simulink model "Md62StEnCtrl"  (R2018b)
settings: Solver=FixedStepDiscrete  StartTime=0.0  StopTime=10.0  RelTol=1e-3
undefined symbols (not defined in the file or in its folder): data, KeSMSuFirstRwStBackPosDelta_Val, KeSMSuThrdRwCushFoldPosDelta_Val, KeSMSwAcsMd30PassStFldUpwdDnwdPos1_Val, KeSMSwAcsMd30PassStFrwdBkwdPos1_Val, KeSMSwAcsMd31PassStBkReclnUpwdDnwdPos1_Val, KeSMSwSeatBkLimitPos_Val, KeSMSwSeatBkLimitPosDelt_Val, PassStBkReclnEn_Clear, PassStBkReclnEn_Set, PassStCshnFldEn_Clear, PassStCshnFldEn_Set, PassStFwdBkwdEn_Clear, PassStFwdBkwdEn_Set, SecRwLtStBkReclnEn_Clear, SecRwLtStBkReclnEn_Set, SecRwLtStFwdBkwdEn_Clear, SecRwLtStFwdBkwdEn_Set, SecRwLtStLgrstInwdOtwdEn_Clear, SecRwLtStLgrstInwdOtwdEn_Set, SecRwLtStLgrstUpwdDnwdEn_Clear, SecRwLtStLgrstUpwdDnwdEn_Set, SecRwRtStBkReclnEn_Clear, SecRwRtStBkReclnEn_Set, SecRwRtStFwdBkwdEn_Clear, SecRwRtStFwdBkwdEn_Set, SecRwRtStLgrstInwdOtwdEn_Clear, SecRwRtStLgrstInwdOtwdEn_Set, SecRwRtStLgrstUpwdDnwdEn_Clear, SecRwRtStLgrstUpwdDnwdEn_Set, ThdRwLtStBkReclnEn_Clear, ThdRwLtStBkReclnEn_Set, ThdRwLtStCshnFldEn_Clear, ThdRwLtStCshnFldEn_Set, ThdRwLtStFwdBkwdEn_Clear, ThdRwLtStFwdBkwdEn_Set, ThdRwRtStBkReclnEn_Clear, ThdRwRtStBkReclnEn_Set, ThdRwRtStCshnFldEn_Clear, ThdRwRtStCshnFldEn_Set, ThdRwRtStFwdBkwdEn_Clear, ThdRwRtStFwdBkwdEn_Set, ZeroLEn_Clear, ZeroLEn_Set, ZeroREn_Clear, ZeroREn_Set
libraries: simulink x1
(part 1 of 3)
settings Model: Creator=sn2xws  LastModifiedBy=sn55gm
settings Model: ModifiedHistory=|
  | 25.7.8 V3.13.0 新增Md62
  | 25.7.14 V3.13.1 TrgtPosZone 选择bit位更新
  | 25.7.25 V1.13.3  记忆位置为展开状态，VCU调用mode 61，三排前后电机应和靠背电机一起驱动到目标位置
settings DataIOCC: SaveFormat=StructureWithTime
settings OptimizationCC: DefaultParameterBehavior=Inlined  EnhancedBackFolding=on  PassReuseOutputArgsAs=Individual arguments  ZeroExternalMemoryAtStartup=off  ZeroInternalMemoryAtStartup=off  OptimizeBlockOrder=speed  DifferentSizesBufferReuse=on  OptimizationCustomize=off
settings DebuggingCC: ParameterTunabilityLossMsg=error
settings SFSimCC: MATLABDynamicMemAlloc=off
settings RTWCC: SystemTargetFile=autosar.tlc  GenCodeOnly=on  TemplateMakefile=ert_default_tmf  Description=AUTOSAR  GenerateReport=on  IncludeHyperlinkInReport=on  LaunchReport=on  GenerateTraceInfo=on  GenerateTraceReport=on  GenerateTraceReportSl=on  GenerateTraceReportSf=on  GenerateTraceReportEml=on
settings CodeAppCC: ForceParamTrailComments=on  IgnoreCustomStorageClasses=off  OperatorAnnotations=on  SimulinkDataObjDesc=on  SFDataObjDesc=on  InsertBlockDesc=on
settings STFCustomTargetCC: TargetLangStandard=C99 (ISO)  MultiwordLength=256  ParMdlRefBuildCompliant=on  CompOptLevelCompliant=on  IncludeMdlTerminateFcn=off  CombineOutputUpdateFcns=on  SuppressErrorStatus=on  ERTCustomFileBanners=on  SupportNonFinite=off  SupportComplex=off  SupportContinuousTime=off  SupportNonInlinedSFcns=off  RemoveResetFunc=on  MATLABClassNameForMDSCustomization=Simulink.SoftwareTarget.ERTCustomization  AutosarCompliant=on  UseToolchainInfoCompliant=on  LookupTableObjectStructAxisOrder=2,1,3,4,...  LUTObjectStructOrderEvenSpacing=Size,Table,Breakpoints  SystemTargetFile=autosar.tlc
settings ERTTargetCC: TargetLangStandard=C99 (ISO)  ConcurrentExecutionCompliant=off  IncludeMdlTerminateFcn=off  SuppressErrorStatus=on  SupportNonFinite=off  SupportComplex=off  ModelStepFunctionPrototypeControlCompliant=off  CPPClassGenCompliant=off  AutosarCompliant=on  LookupTableObjectStructAxisOrder=2,1,3,4,...  LUTObjectStructOrderEvenSpacing=Size,Table,Breakpoints  InlinedParameterPlacement=NonHierarchical  ERTCustomFileTemplate=example_file_process.tlc  ERTFilePackagingFormat=Compact

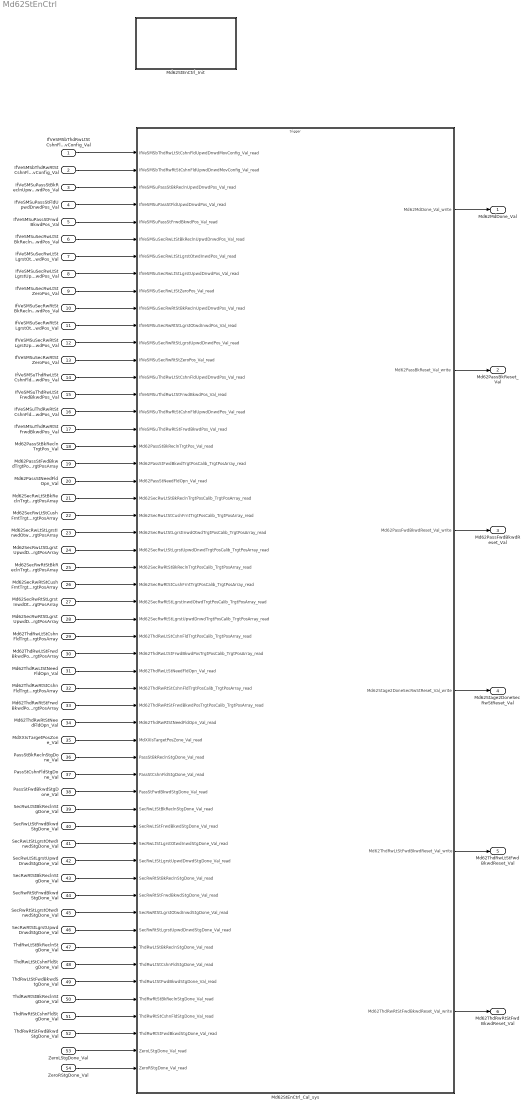
== system Md62StEnCtrl ==
  IfVeSMSbThdRwLtStCshnFldUpwdDnwdMovConfig_Val : Inport  OutDataTypeStr=boolean  PortDimensions=1
  IfVeSMSbThdRwRtStCshnFldUpwdDnwdMovConfig_Val : Inport  Port=2  OutDataTypeStr=boolean  PortDimensions=1
  IfVeSMSuPassStBkReclnUpwdDnwdPos_Val : Inport  Port=3  OutDataTypeStr=uint16  PortDimensions=1
  IfVeSMSuPassStFldUpwdDnwdPos_Val : Inport  Port=4  OutDataTypeStr=uint16  PortDimensions=1
  IfVeSMSuPassStFrwdBkwdPos_Val : Inport  Port=5  OutDataTypeStr=uint16  PortDimensions=1
  IfVeSMSuSecRwLtStBkReclnUpwdDnwdPos_Val : Inport  Port=6  OutDataTypeStr=uint16  PortDimensions=1
  IfVeSMSuSecRwLtStLgrstOtwdInwdPos_Val : Inport  Port=7  OutDataTypeStr=uint16  PortDimensions=1
  IfVeSMSuSecRwLtStLgrstUpwdDnwdPos_Val : Inport  Port=8  OutDataTypeStr=uint16  PortDimensions=1
  IfVeSMSuSecRwLtStZeroPos_Val : Inport  Port=9  OutDataTypeStr=uint16  PortDimensions=1
  IfVeSMSuSecRwRtStBkReclnUpwdDnwdPos_Val : Inport  Port=10  OutDataTypeStr=uint16  PortDimensions=1
  IfVeSMSuSecRwRtStLgrstOtwdInwdPos_Val : Inport  Port=11  OutDataTypeStr=uint16  PortDimensions=1
  IfVeSMSuSecRwRtStLgrstUpwdDnwdPos_Val : Inport  Port=12  OutDataTypeStr=uint16  PortDimensions=1
  IfVeSMSuSecRwRtStZeroPos_Val : Inport  Port=13  OutDataTypeStr=uint16  PortDimensions=1
  IfVeSMSuThdRwLtStCshnFldUpwdDnwdPos_Val : Inport  Port=14  OutDataTypeStr=uint16  PortDimensions=1
  IfVeSMSuThdRwLtStFrwdBkwdPos_Val : Inport  Port=15  OutDataTypeStr=uint16  PortDimensions=1
  IfVeSMSuThdRwRtStCshnFldUpwdDnwdPos_Val : Inport  Port=16  OutDataTypeStr=uint16  PortDimensions=1
  IfVeSMSuThdRwRtStFrwdBkwdPos_Val : Inport  Port=17  OutDataTypeStr=uint16  PortDimensions=1
  Md62PassStBkReclnTrgtPos_Val : Inport  Port=18  OutDataTypeStr=uint16  PortDimensions=1
  Md62PassStFwdBkwdTrgtPosCalib_TrgtPosArray : Inport  Description=|  Port=19  OutDataTypeStr=uint16  PortDimensions=3
      | 0:Pos
      | 1:Max
      | 2:Min
  Md62PassStNeedFldOpn_Val : Inport  Port=20  OutDataTypeStr=boolean  PortDimensions=1
  Md62SecRwLtStBkReclnTrgtPosCalib_TrgtPosArray : Inport  Description=|  Port=21  OutDataTypeStr=uint16  PortDimensions=3
      | 0:Pos
      | 1:Max
      | 2:Min
  Md62SecRwLtStCushFrntTrgtPosCalib_TrgtPosArray : Inport  Description=|  Port=22  OutDataTypeStr=uint16  PortDimensions=3
      | 0:Pos
      | 1:Max
      | 2:Min
  Md62SecRwLtStLgrstInwdOtwdTrgtPosCalib_TrgtPosArray : Inport  Description=|  Port=23  OutDataTypeStr=uint16  PortDimensions=3
      | 0:Pos
      | 1:Max
      | 2:Min
  Md62SecRwLtStLgrstUpwdDnwdTrgtPosCalib_TrgtPosArray : Inport  Description=|  Port=24  OutDataTypeStr=uint16  PortDimensions=3
      | 0:Pos
      | 1:Max
      | 2:Min
  Md62SecRwRtStBkReclnTrgtPosCalib_TrgtPosArray : Inport  Description=|  Port=25  OutDataTypeStr=uint16  PortDimensions=3
      | 0:Pos
      | 1:Max
      | 2:Min
  Md62SecRwRtStCushFrntTrgtPosCalib_TrgtPosArray : Inport  Description=|  Port=26  OutDataTypeStr=uint16  PortDimensions=3
      | 0:Pos
      | 1:Max
      | 2:Min
  Md62SecRwRtStLgrstInwdOtwdTrgtPosCalib_TrgtPosArray : Inport  Description=|  Port=27  OutDataTypeStr=uint16  PortDimensions=3
      | 0:Pos
      | 1:Max
      | 2:Min
  Md62SecRwRtStLgrstUpwdDnwdTrgtPosCalib_TrgtPosArray : Inport  Description=|  Port=28  OutDataTypeStr=uint16  PortDimensions=3
      | 0:Pos
      | 1:Max
      | 2:Min
  Md62ThdRwLtStCshnFldTrgtPosCalib_TrgtPosArray : Inport  Description=|  Port=29  OutDataTypeStr=uint16  PortDimensions=3
      | 0:Pos
      | 1:Max
      | 2:Min
  Md62ThdRwLtStFrwdBkwdPosTrgtPosCalib_TrgtPosArray : Inport  Description=|  Port=30  OutDataTypeStr=uint16  PortDimensions=3
      | 0:Pos
      | 1:Max
      | 2:Min
  Md62ThdRwLtStNeedFldOpn_Val : Inport  Port=31  OutDataTypeStr=boolean  PortDimensions=1
  Md62ThdRwRtStCshnFldTrgtPosCalib_TrgtPosArray : Inport  Description=|  Port=32  OutDataTypeStr=uint16  PortDimensions=3
      | 0:Pos
      | 1:Max
      | 2:Min
  Md62ThdRwRtStFrwdBkwdPosTrgtPosCalib_TrgtPosArray : Inport  Description=|  Port=33  OutDataTypeStr=uint16  PortDimensions=3
      | 0:Pos
      | 1:Max
      | 2:Min
  Md62ThdRwRtStNeedFldOpn_Val : Inport  Port=34  OutDataTypeStr=boolean  PortDimensions=1
  MdXXIsTargetPosZone_Val : Inport  Port=35  OutDataTypeStr=uint32  PortDimensions=1
  PassStBkReclnStgDone_Val : Inport  Port=36  OutDataTypeStr=boolean  PortDimensions=1
  PassStCshnFldStgDone_Val : Inport  Port=37  OutDataTypeStr=boolean  PortDimensions=1
  PassStFwdBkwdStgDone_Val : Inport  Port=38  OutDataTypeStr=boolean  PortDimensions=1
  SecRwLtStBkReclnStgDone_Val : Inport  Port=39  OutDataTypeStr=boolean  PortDimensions=1
  SecRwLtStFrwdBkwdStgDone_Val : Inport  Port=40  OutDataTypeStr=boolean  PortDimensions=1
  SecRwLtStLgrstOtwdInwdStgDone_Val : Inport  Port=41  OutDataTypeStr=boolean  PortDimensions=1
  SecRwLtStLgrstUpwdDnwdStgDone_Val : Inport  Port=42  OutDataTypeStr=boolean  PortDimensions=1
  SecRwRtStBkReclnStgDone_Val : Inport  Port=43  OutDataTypeStr=boolean  PortDimensions=1
  SecRwRtStFrwdBkwdStgDone_Val : Inport  Port=44  OutDataTypeStr=boolean  PortDimensions=1
  SecRwRtStLgrstOtwdInwdStgDone_Val : Inport  Port=45  OutDataTypeStr=boolean  PortDimensions=1
  SecRwRtStLgrstUpwdDnwdStgDone_Val : Inport  Port=46  OutDataTypeStr=boolean  PortDimensions=1
  ThdRwLtStBkReclnStgDone_Val : Inport  Port=47  OutDataTypeStr=boolean  PortDimensions=1
  ThdRwLtStCshnFldStgDone_Val : Inport  Port=48  OutDataTypeStr=boolean  PortDimensions=1
  ThdRwLtStFwdBkwdStgDone_Val : Inport  Port=49  OutDataTypeStr=boolean  PortDimensions=1
  ThdRwRtStBkReclnStgDone_Val : Inport  Port=50  OutDataTypeStr=boolean  PortDimensions=1
  ThdRwRtStCshnFldStgDone_Val : Inport  Port=51  OutDataTypeStr=boolean  PortDimensions=1
  ThdRwRtStFwdBkwdStgDone_Val : Inport  Port=52  OutDataTypeStr=boolean  PortDimensions=1
  ZeroLStgDone_Val : Inport  Port=53  OutDataTypeStr=boolean  PortDimensions=1
  ZeroRStgDone_Val : Inport  Port=54  OutDataTypeStr=boolean  PortDimensions=1
  Md62StEnCtrl_Cal_sys : Subsystem
  Md62StEnCtrl_Init : Subsystem
  Md62MdDone_Val : Outport  OutDataTypeStr=uint8  PortDimensions=1
  Md62PassBkReset_Val : Outport  Port=2  OutDataTypeStr=boolean  PortDimensions=1
  Md62PassFwdBkwdReset_Val : Outport  Port=3  OutDataTypeStr=boolean  PortDimensions=1
  Md62Stage2DoneSecRwStReset_Val : Outport  Port=4  OutDataTypeStr=boolean  PortDimensions=1
  Md62ThdRwLtStFwdBkwdReset_Val : Outport  Port=5  OutDataTypeStr=boolean  PortDimensions=1
  Md62ThdRwRtStFwdBkwdReset_Val : Outport  Port=6  OutDataTypeStr=boolean  PortDimensions=1
  wires:
  IfVeSMSbThdRwLtStCshnFldUpwdDnwdMovConfig_Val/1 -> Md62StEnCtrl_Cal_sys/1(IfVeSMSbThdRwLtStCshnFldUpwdDnwdMovConfig_Val_read)
  IfVeSMSbThdRwRtStCshnFldUpwdDnwdMovConfig_Val/1 -> Md62StEnCtrl_Cal_sys/2(IfVeSMSbThdRwRtStCshnFldUpwdDnwdMovConfig_Val_read)
  IfVeSMSuPassStBkReclnUpwdDnwdPos_Val/1 -> Md62StEnCtrl_Cal_sys/3(IfVeSMSuPassStBkReclnUpwdDnwdPos_Val_read)
  IfVeSMSuPassStFldUpwdDnwdPos_Val/1 -> Md62StEnCtrl_Cal_sys/4(IfVeSMSuPassStFldUpwdDnwdPos_Val_read)
  IfVeSMSuPassStFrwdBkwdPos_Val/1 -> Md62StEnCtrl_Cal_sys/5(IfVeSMSuPassStFrwdBkwdPos_Val_read)
  IfVeSMSuSecRwLtStBkReclnUpwdDnwdPos_Val/1 -> Md62StEnCtrl_Cal_sys/6(IfVeSMSuSecRwLtStBkReclnUpwdDnwdPos_Val_read)
  IfVeSMSuSecRwLtStLgrstOtwdInwdPos_Val/1 -> Md62StEnCtrl_Cal_sys/7(IfVeSMSuSecRwLtStLgrstOtwdInwdPos_Val_read)
  IfVeSMSuSecRwLtStLgrstUpwdDnwdPos_Val/1 -> Md62StEnCtrl_Cal_sys/8(IfVeSMSuSecRwLtStLgrstUpwdDnwdPos_Val_read)
  IfVeSMSuSecRwLtStZeroPos_Val/1 -> Md62StEnCtrl_Cal_sys/9(IfVeSMSuSecRwLtStZeroPos_Val_read)
  IfVeSMSuSecRwRtStBkReclnUpwdDnwdPos_Val/1 -> Md62StEnCtrl_Cal_sys/10(IfVeSMSuSecRwRtStBkReclnUpwdDnwdPos_Val_read)
  IfVeSMSuSecRwRtStLgrstOtwdInwdPos_Val/1 -> Md62StEnCtrl_Cal_sys/11(IfVeSMSuSecRwRtStLgrstOtwdInwdPos_Val_read)
  IfVeSMSuSecRwRtStLgrstUpwdDnwdPos_Val/1 -> Md62StEnCtrl_Cal_sys/12(IfVeSMSuSecRwRtStLgrstUpwdDnwdPos_Val_read)
  IfVeSMSuSecRwRtStZeroPos_Val/1 -> Md62StEnCtrl_Cal_sys/13(IfVeSMSuSecRwRtStZeroPos_Val_read)
  IfVeSMSuThdRwLtStCshnFldUpwdDnwdPos_Val/1 -> Md62StEnCtrl_Cal_sys/14(IfVeSMSuThdRwLtStCshnFldUpwdDnwdPos_Val_read)
  IfVeSMSuThdRwLtStFrwdBkwdPos_Val/1 -> Md62StEnCtrl_Cal_sys/15(IfVeSMSuThdRwLtStFrwdBkwdPos_Val_read)
  IfVeSMSuThdRwRtStCshnFldUpwdDnwdPos_Val/1 -> Md62StEnCtrl_Cal_sys/16(IfVeSMSuThdRwRtStCshnFldUpwdDnwdPos_Val_read)
  IfVeSMSuThdRwRtStFrwdBkwdPos_Val/1 -> Md62StEnCtrl_Cal_sys/17(IfVeSMSuThdRwRtStFrwdBkwdPos_Val_read)
  Md62PassStBkReclnTrgtPos_Val/1 -> Md62StEnCtrl_Cal_sys/18(Md62PassStBkReclnTrgtPos_Val_read)
  Md62PassStFwdBkwdTrgtPosCalib_TrgtPosArray/1 -> Md62StEnCtrl_Cal_sys/19(Md62PassStFwdBkwdTrgtPosCalib_TrgtPosArray_read)
  Md62PassStNeedFldOpn_Val/1 -> Md62StEnCtrl_Cal_sys/20(Md62PassStNeedFldOpn_Val_read)
  Md62SecRwLtStBkReclnTrgtPosCalib_TrgtPosArray/1 -> Md62StEnCtrl_Cal_sys/21(Md62SecRwLtStBkReclnTrgtPosCalib_TrgtPosArray_read)
  Md62SecRwLtStCushFrntTrgtPosCalib_TrgtPosArray/1 -> Md62StEnCtrl_Cal_sys/22(Md62SecRwLtStCushFrntTrgtPosCalib_TrgtPosArray_read)
  Md62SecRwLtStLgrstInwdOtwdTrgtPosCalib_TrgtPosArray/1 -> Md62StEnCtrl_Cal_sys/23(Md62SecRwLtStLgrstInwdOtwdTrgtPosCalib_TrgtPosArray_read)
  Md62SecRwLtStLgrstUpwdDnwdTrgtPosCalib_TrgtPosArray/1 -> Md62StEnCtrl_Cal_sys/24(Md62SecRwLtStLgrstUpwdDnwdTrgtPosCalib_TrgtPosArray_read)
  Md62SecRwRtStBkReclnTrgtPosCalib_TrgtPosArray/1 -> Md62StEnCtrl_Cal_sys/25(Md62SecRwRtStBkReclnTrgtPosCalib_TrgtPosArray_read)
  Md62SecRwRtStCushFrntTrgtPosCalib_TrgtPosArray/1 -> Md62StEnCtrl_Cal_sys/26(Md62SecRwRtStCushFrntTrgtPosCalib_TrgtPosArray_read)
  Md62SecRwRtStLgrstInwdOtwdTrgtPosCalib_TrgtPosArray/1 -> Md62StEnCtrl_Cal_sys/27(Md62SecRwRtStLgrstInwdOtwdTrgtPosCalib_TrgtPosArray_read)
  Md62SecRwRtStLgrstUpwdDnwdTrgtPosCalib_TrgtPosArray/1 -> Md62StEnCtrl_Cal_sys/28(Md62SecRwRtStLgrstUpwdDnwdTrgtPosCalib_TrgtPosArray_read)
  Md62ThdRwLtStCshnFldTrgtPosCalib_TrgtPosArray/1 -> Md62StEnCtrl_Cal_sys/29(Md62ThdRwLtStCshnFldTrgtPosCalib_TrgtPosArray_read)
  Md62ThdRwLtStFrwdBkwdPosTrgtPosCalib_TrgtPosArray/1 -> Md62StEnCtrl_Cal_sys/30(Md62ThdRwLtStFrwdBkwdPosTrgtPosCalib_TrgtPosArray_read)
  Md62ThdRwLtStNeedFldOpn_Val/1 -> Md62StEnCtrl_Cal_sys/31(Md62ThdRwLtStNeedFldOpn_Val_read)
  Md62ThdRwRtStCshnFldTrgtPosCalib_TrgtPosArray/1 -> Md62StEnCtrl_Cal_sys/32(Md62ThdRwRtStCshnFldTrgtPosCalib_TrgtPosArray_read)
  Md62ThdRwRtStFrwdBkwdPosTrgtPosCalib_TrgtPosArray/1 -> Md62StEnCtrl_Cal_sys/33(Md62ThdRwRtStFrwdBkwdPosTrgtPosCalib_TrgtPosArray_read)
  Md62ThdRwRtStNeedFldOpn_Val/1 -> Md62StEnCtrl_Cal_sys/34(Md62ThdRwRtStNeedFldOpn_Val_read)
  MdXXIsTargetPosZone_Val/1 -> Md62StEnCtrl_Cal_sys/35(MdXXIsTargetPosZone_Val_read)
  PassStBkReclnStgDone_Val/1 -> Md62StEnCtrl_Cal_sys/36(PassStBkReclnStgDone_Val_read)
  PassStCshnFldStgDone_Val/1 -> Md62StEnCtrl_Cal_sys/37(PassStCshnFldStgDone_Val_read)
  PassStFwdBkwdStgDone_Val/1 -> Md62StEnCtrl_Cal_sys/38(PassStFwdBkwdStgDone_Val_read)
  SecRwLtStBkReclnStgDone_Val/1 -> Md62StEnCtrl_Cal_sys/39(SecRwLtStBkReclnStgDone_Val_read)
  SecRwLtStFrwdBkwdStgDone_Val/1 -> Md62StEnCtrl_Cal_sys/40(SecRwLtStFrwdBkwdStgDone_Val_read)
  SecRwLtStLgrstOtwdInwdStgDone_Val/1 -> Md62StEnCtrl_Cal_sys/41(SecRwLtStLgrstOtwdInwdStgDone_Val_read)
  SecRwLtStLgrstUpwdDnwdStgDone_Val/1 -> Md62StEnCtrl_Cal_sys/42(SecRwLtStLgrstUpwdDnwdStgDone_Val_read)
  SecRwRtStBkReclnStgDone_Val/1 -> Md62StEnCtrl_Cal_sys/43(SecRwRtStBkReclnStgDone_Val_read)
  SecRwRtStFrwdBkwdStgDone_Val/1 -> Md62StEnCtrl_Cal_sys/44(SecRwRtStFrwdBkwdStgDone_Val_read)
  SecRwRtStLgrstOtwdInwdStgDone_Val/1 -> Md62StEnCtrl_Cal_sys/45(SecRwRtStLgrstOtwdInwdStgDone_Val_read)
  SecRwRtStLgrstUpwdDnwdStgDone_Val/1 -> Md62StEnCtrl_Cal_sys/46(SecRwRtStLgrstUpwdDnwdStgDone_Val_read)
  ThdRwLtStBkReclnStgDone_Val/1 -> Md62StEnCtrl_Cal_sys/47(ThdRwLtStBkReclnStgDone_Val_read)
  ThdRwLtStCshnFldStgDone_Val/1 -> Md62StEnCtrl_Cal_sys/48(ThdRwLtStCshnFldStgDone_Val_read)
  ThdRwLtStFwdBkwdStgDone_Val/1 -> Md62StEnCtrl_Cal_sys/49(ThdRwLtStFwdBkwdStgDone_Val_read)
  ThdRwRtStBkReclnStgDone_Val/1 -> Md62StEnCtrl_Cal_sys/50(ThdRwRtStBkReclnStgDone_Val_read)
  ThdRwRtStCshnFldStgDone_Val/1 -> Md62StEnCtrl_Cal_sys/51(ThdRwRtStCshnFldStgDone_Val_read)
  ThdRwRtStFwdBkwdStgDone_Val/1 -> Md62StEnCtrl_Cal_sys/52(ThdRwRtStFwdBkwdStgDone_Val_read)
  ZeroLStgDone_Val/1 -> Md62StEnCtrl_Cal_sys/53(ZeroLStgDone_Val_read)
  ZeroRStgDone_Val/1 -> Md62StEnCtrl_Cal_sys/54(ZeroRStgDone_Val_read)
  Md62StEnCtrl_Cal_sys/1(Md62MdDone_Val_write) -> Md62MdDone_Val/1
  Md62StEnCtrl_Cal_sys/2(Md62PassBkReset_Val_write) -> Md62PassBkReset_Val/1
  Md62StEnCtrl_Cal_sys/3(Md62PassFwdBkwdReset_Val_write) -> Md62PassFwdBkwdReset_Val/1
  Md62StEnCtrl_Cal_sys/4(Md62Stage2DoneSecRwStReset_Val_write) -> Md62Stage2DoneSecRwStReset_Val/1
  Md62StEnCtrl_Cal_sys/5(Md62ThdRwLtStFwdBkwdReset_Val_write) -> Md62ThdRwLtStFwdBkwdReset_Val/1
  Md62StEnCtrl_Cal_sys/6(Md62ThdRwRtStFwdBkwdReset_Val_write) -> Md62ThdRwRtStFwdBkwdReset_Val/1

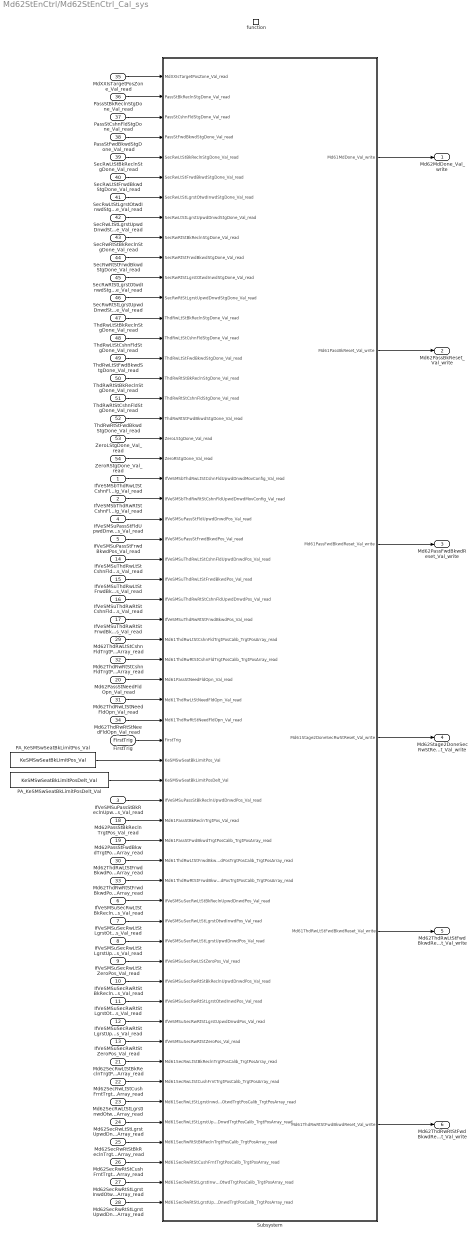
== system Md62StEnCtrl/Md62StEnCtrl_Cal_sys ==
  IfVeSMSbThdRwLtStCshnFldUpwdDnwdMovConfig_Val_read : Inport
  IfVeSMSbThdRwRtStCshnFldUpwdDnwdMovConfig_Val_read : Inport  Port=2
  IfVeSMSuPassStBkReclnUpwdDnwdPos_Val_read : Inport  Port=3
  IfVeSMSuPassStFldUpwdDnwdPos_Val_read : Inport  Port=4
  IfVeSMSuPassStFrwdBkwdPos_Val_read : Inport  Port=5
  IfVeSMSuSecRwLtStBkReclnUpwdDnwdPos_Val_read : Inport  Port=6
  IfVeSMSuSecRwLtStLgrstOtwdInwdPos_Val_read : Inport  Port=7
  IfVeSMSuSecRwLtStLgrstUpwdDnwdPos_Val_read : Inport  Port=8
  IfVeSMSuSecRwLtStZeroPos_Val_read : Inport  Port=9
  IfVeSMSuSecRwRtStBkReclnUpwdDnwdPos_Val_read : Inport  Port=10
  IfVeSMSuSecRwRtStLgrstOtwdInwdPos_Val_read : Inport  Port=11
  IfVeSMSuSecRwRtStLgrstUpwdDnwdPos_Val_read : Inport  Port=12
  IfVeSMSuSecRwRtStZeroPos_Val_read : Inport  Port=13
  IfVeSMSuThdRwLtStCshnFldUpwdDnwdPos_Val_read : Inport  Port=14
  IfVeSMSuThdRwLtStFrwdBkwdPos_Val_read : Inport  Port=15
  IfVeSMSuThdRwRtStCshnFldUpwdDnwdPos_Val_read : Inport  Port=16
  IfVeSMSuThdRwRtStFrwdBkwdPos_Val_read : Inport  Port=17
  Md62PassStBkReclnTrgtPos_Val_read : Inport  Port=18
  Md62PassStFwdBkwdTrgtPosCalib_TrgtPosArray_read : Inport  Port=19
  Md62PassStNeedFldOpn_Val_read : Inport  Port=20
  Md62SecRwLtStBkReclnTrgtPosCalib_TrgtPosArray_read : Inport  Port=21
  Md62SecRwLtStCushFrntTrgtPosCalib_TrgtPosArray_read : Inport  Port=22
  Md62SecRwLtStLgrstInwdOtwdTrgtPosCalib_TrgtPosArray_read : Inport  Port=23
  Md62SecRwLtStLgrstUpwdDnwdTrgtPosCalib_TrgtPosArray_read : Inport  Port=24
  Md62SecRwRtStBkReclnTrgtPosCalib_TrgtPosArray_read : Inport  Port=25
  Md62SecRwRtStCushFrntTrgtPosCalib_TrgtPosArray_read : Inport  Port=26
  Md62SecRwRtStLgrstInwdOtwdTrgtPosCalib_TrgtPosArray_read : Inport  Port=27
  Md62SecRwRtStLgrstUpwdDnwdTrgtPosCalib_TrgtPosArray_read : Inport  Port=28
  Md62ThdRwLtStCshnFldTrgtPosCalib_TrgtPosArray_read : Inport  Port=29
  Md62ThdRwLtStFrwdBkwdPosTrgtPosCalib_TrgtPosArray_read : Inport  Port=30
  Md62ThdRwLtStNeedFldOpn_Val_read : Inport  Port=31
  Md62ThdRwRtStCshnFldTrgtPosCalib_TrgtPosArray_read : Inport  Port=32
  Md62ThdRwRtStFrwdBkwdPosTrgtPosCalib_TrgtPosArray_read : Inport  Port=33
  Md62ThdRwRtStNeedFldOpn_Val_read : Inport  Port=34
  MdXXIsTargetPosZone_Val_read : Inport  Port=35
  PassStBkReclnStgDone_Val_read : Inport  Port=36
  PassStCshnFldStgDone_Val_read : Inport  Port=37
  PassStFwdBkwdStgDone_Val_read : Inport  Port=38
  SecRwLtStBkReclnStgDone_Val_read : Inport  Port=39
  SecRwLtStFrwdBkwdStgDone_Val_read : Inport  Port=40
  SecRwLtStLgrstOtwdInwdStgDone_Val_read : Inport  Port=41
  SecRwLtStLgrstUpwdDnwdStgDone_Val_read : Inport  Port=42
  SecRwRtStBkReclnStgDone_Val_read : Inport  Port=43
  SecRwRtStFrwdBkwdStgDone_Val_read : Inport  Port=44
  SecRwRtStLgrstOtwdInwdStgDone_Val_read : Inport  Port=45
  SecRwRtStLgrstUpwdDnwdStgDone_Val_read : Inport  Port=46
  ThdRwLtStBkReclnStgDone_Val_read : Inport  Port=47
  ThdRwLtStCshnFldStgDone_Val_read : Inport  Port=48
  ThdRwLtStFwdBkwdStgDone_Val_read : Inport  Port=49
  ThdRwRtStBkReclnStgDone_Val_read : Inport  Port=50
  ThdRwRtStCshnFldStgDone_Val_read : Inport  Port=51
  ThdRwRtStFwdBkwdStgDone_Val_read : Inport  Port=52
  ZeroLStgDone_Val_read : Inport  Port=53
  ZeroRStgDone_Val_read : Inport  Port=54
  function : TriggerPort  TriggerType=function-call  IsSimulinkFunction=on  FunctionName=Md62StEnCtrl_Cal  VariantControl=(inherit)
  PA_KeSMSwSeatBkLimitPosDelt_Val : Constant  Value=KeSMSwSeatBkLimitPosDelt_Val
  PA_KeSMSwSeatBkLimitPos_Val : Constant  Value=KeSMSwSeatBkLimitPos_Val
  Subsystem : Subsystem
  FirstTrig : ArgIn  OutDataTypeStr=boolean  ArgumentName=FirstTrig
  Md62MdDone_Val_write : Outport
      settings: EnsureOutportIsVirtual=on
  Md62PassBkReset_Val_write : Outport  Port=2
      settings: EnsureOutportIsVirtual=on
  Md62PassFwdBkwdReset_Val_write : Outport  Port=3
      settings: EnsureOutportIsVirtual=on
  Md62Stage2DoneSecRwStReset_Val_write : Outport  Port=4
      settings: EnsureOutportIsVirtual=on
  Md62ThdRwLtStFwdBkwdReset_Val_write : Outport  Port=5
      settings: EnsureOutportIsVirtual=on
  Md62ThdRwRtStFwdBkwdReset_Val_write : Outport  Port=6
      settings: EnsureOutportIsVirtual=on
  wires:
  Subsystem/1(Md61MdDone_Val_write) -> Md62MdDone_Val_write/1
  Subsystem/2(Md61PassBkReset_Val_write) -> Md62PassBkReset_Val_write/1
  Subsystem/3(Md61PassFwdBkwdReset_Val_write) -> Md62PassFwdBkwdReset_Val_write/1
  Subsystem/4(Md61Stage2DoneSecRwStReset_Val_write) -> Md62Stage2DoneSecRwStReset_Val_write/1
  Subsystem/5(Md61ThdRwLtStFwdBkwdReset_Val_write) -> Md62ThdRwLtStFwdBkwdReset_Val_write/1
  Subsystem/6(Md61ThdRwRtStFwdBkwdReset_Val_write) -> Md62ThdRwRtStFwdBkwdReset_Val_write/1
  ZeroLStgDone_Val_read/1 -> Subsystem/19(ZeroLStgDone_Val_read)
  ZeroRStgDone_Val_read/1 -> Subsystem/20(ZeroRStgDone_Val_read)
  MdXXIsTargetPosZone_Val_read/1 -> Subsystem/1(MdXXIsTargetPosZone_Val_read)
  PassStBkReclnStgDone_Val_read/1 -> Subsystem/2(PassStBkReclnStgDone_Val_read)
  PassStCshnFldStgDone_Val_read/1 -> Subsystem/3(PassStCshnFldStgDone_Val_read)
  PassStFwdBkwdStgDone_Val_read/1 -> Subsystem/4(PassStFwdBkwdStgDone_Val_read)
  SecRwLtStBkReclnStgDone_Val_read/1 -> Subsystem/5(SecRwLtStBkReclnStgDone_Val_read)
  SecRwLtStFrwdBkwdStgDone_Val_read/1 -> Subsystem/6(SecRwLtStFrwdBkwdStgDone_Val_read)
  SecRwLtStLgrstOtwdInwdStgDone_Val_read/1 -> Subsystem/7(SecRwLtStLgrstOtwdInwdStgDone_Val_read)
  SecRwLtStLgrstUpwdDnwdStgDone_Val_read/1 -> Subsystem/8(SecRwLtStLgrstUpwdDnwdStgDone_Val_read)
  SecRwRtStBkReclnStgDone_Val_read/1 -> Subsystem/9(SecRwRtStBkReclnStgDone_Val_read)
  SecRwRtStFrwdBkwdStgDone_Val_read/1 -> Subsystem/10(SecRwRtStFrwdBkwdStgDone_Val_read)
  SecRwRtStLgrstOtwdInwdStgDone_Val_read/1 -> Subsystem/11(SecRwRtStLgrstOtwdInwdStgDone_Val_read)
  SecRwRtStLgrstUpwdDnwdStgDone_Val_read/1 -> Subsystem/12(SecRwRtStLgrstUpwdDnwdStgDone_Val_read)
  ThdRwLtStBkReclnStgDone_Val_read/1 -> Subsystem/13(ThdRwLtStBkReclnStgDone_Val_read)
  ThdRwLtStCshnFldStgDone_Val_read/1 -> Subsystem/14(ThdRwLtStCshnFldStgDone_Val_read)
  ThdRwLtStFwdBkwdStgDone_Val_read/1 -> Subsystem/15(ThdRwLtStFwdBkwdStgDone_Val_read)
  ThdRwRtStBkReclnStgDone_Val_read/1 -> Subsystem/16(ThdRwRtStBkReclnStgDone_Val_read)
  ThdRwRtStCshnFldStgDone_Val_read/1 -> Subsystem/17(ThdRwRtStCshnFldStgDone_Val_read)
  ThdRwRtStFwdBkwdStgDone_Val_read/1 -> Subsystem/18(ThdRwRtStFwdBkwdStgDone_Val_read)
  IfVeSMSbThdRwLtStCshnFldUpwdDnwdMovConfig_Val_read/1 -> Subsystem/21(IfVeSMSbThdRwLtStCshnFldUpwdDnwdMovConfig_Val_read)
  IfVeSMSbThdRwRtStCshnFldUpwdDnwdMovConfig_Val_read/1 -> Subsystem/22(IfVeSMSbThdRwRtStCshnFldUpwdDnwdMovConfig_Val_read)
  IfVeSMSuPassStFrwdBkwdPos_Val_read/1 -> Subsystem/24(IfVeSMSuPassStFrwdBkwdPos_Val_read)
  IfVeSMSuThdRwLtStFrwdBkwdPos_Val_read/1 -> Subsystem/26(IfVeSMSuThdRwLtStFrwdBkwdPos_Val_read)
  IfVeSMSuThdRwRtStFrwdBkwdPos_Val_read/1 -> Subsystem/28(IfVeSMSuThdRwRtStFrwdBkwdPos_Val_read)
  Md62ThdRwLtStCshnFldTrgtPosCalib_TrgtPosArray_read/1 -> Subsystem/29(Md61ThdRwLtStCshnFldTrgtPosCalib_TrgtPosArray_read)
  Md62ThdRwRtStCshnFldTrgtPosCalib_TrgtPosArray_read/1 -> Subsystem/30(Md61ThdRwRtStCshnFldTrgtPosCalib_TrgtPosArray_read)
  Md62ThdRwLtStNeedFldOpn_Val_read/1 -> Subsystem/32(Md61ThdRwLtStNeedFldOpn_Val_read)
  Md62ThdRwRtStNeedFldOpn_Val_read/1 -> Subsystem/33(Md61ThdRwRtStNeedFldOpn_Val_read)
  Md62PassStNeedFldOpn_Val_read/1 -> Subsystem/31(Md61PassStNeedFldOpn_Val_read)
  FirstTrig/1 -> Subsystem/34(FirstTrig)
  PA_KeSMSwSeatBkLimitPos_Val/1 -> Subsystem/35(KeSMSwSeatBkLimitPos_Val)
  PA_KeSMSwSeatBkLimitPosDelt_Val/1 -> Subsystem/36(KeSMSwSeatBkLimitPosDelt_Val)
  Md62PassStBkReclnTrgtPos_Val_read/1 -> Subsystem/38(Md61PassStBkReclnTrgtPos_Val_read)
  Md62PassStFwdBkwdTrgtPosCalib_TrgtPosArray_read/1 -> Subsystem/39(Md61PassStFwdBkwdTrgtPosCalib_TrgtPosArray_read)
  Md62ThdRwLtStFrwdBkwdPosTrgtPosCalib_TrgtPosArray_read/1 -> Subsystem/40(Md61ThdRwLtStFrwdBkwdPosTrgtPosCalib_TrgtPosArray_read)
  Md62ThdRwRtStFrwdBkwdPosTrgtPosCalib_TrgtPosArray_read/1 -> Subsystem/41(Md61ThdRwRtStFrwdBkwdPosTrgtPosCalib_TrgtPosArray_read)
  IfVeSMSuPassStFldUpwdDnwdPos_Val_read/1 -> Subsystem/23(IfVeSMSuPassStFldUpwdDnwdPos_Val_read)
  IfVeSMSuPassStBkReclnUpwdDnwdPos_Val_read/1 -> Subsystem/37(IfVeSMSuPassStBkReclnUpwdDnwdPos_Val_read)
  IfVeSMSuThdRwLtStCshnFldUpwdDnwdPos_Val_read/1 -> Subsystem/25(IfVeSMSuThdRwLtStCshnFldUpwdDnwdPos_Val_read)
  IfVeSMSuThdRwRtStCshnFldUpwdDnwdPos_Val_read/1 -> Subsystem/27(IfVeSMSuThdRwRtStCshnFldUpwdDnwdPos_Val_read)
  IfVeSMSuSecRwLtStBkReclnUpwdDnwdPos_Val_read/1 -> Subsystem/42(IfVeSMSuSecRwLtStBkReclnUpwdDnwdPos_Val_read)
  IfVeSMSuSecRwLtStLgrstOtwdInwdPos_Val_read/1 -> Subsystem/43(IfVeSMSuSecRwLtStLgrstOtwdInwdPos_Val_read)
  IfVeSMSuSecRwLtStLgrstUpwdDnwdPos_Val_read/1 -> Subsystem/44(IfVeSMSuSecRwLtStLgrstUpwdDnwdPos_Val_read)
  IfVeSMSuSecRwLtStZeroPos_Val_read/1 -> Subsystem/45(IfVeSMSuSecRwLtStZeroPos_Val_read)
  IfVeSMSuSecRwRtStBkReclnUpwdDnwdPos_Val_read/1 -> Subsystem/46(IfVeSMSuSecRwRtStBkReclnUpwdDnwdPos_Val_read)
  IfVeSMSuSecRwRtStLgrstOtwdInwdPos_Val_read/1 -> Subsystem/47(IfVeSMSuSecRwRtStLgrstOtwdInwdPos_Val_read)
  IfVeSMSuSecRwRtStLgrstUpwdDnwdPos_Val_read/1 -> Subsystem/48(IfVeSMSuSecRwRtStLgrstUpwdDnwdPos_Val_read)
  IfVeSMSuSecRwRtStZeroPos_Val_read/1 -> Subsystem/49(IfVeSMSuSecRwRtStZeroPos_Val_read)
  Md62SecRwLtStBkReclnTrgtPosCalib_TrgtPosArray_read/1 -> Subsystem/50(Md61SecRwLtStBkReclnTrgtPosCalib_TrgtPosArray_read)
  Md62SecRwLtStCushFrntTrgtPosCalib_TrgtPosArray_read/1 -> Subsystem/51(Md61SecRwLtStCushFrntTrgtPosCalib_TrgtPosArray_read)
  Md62SecRwLtStLgrstInwdOtwdTrgtPosCalib_TrgtPosArray_read/1 -> Subsystem/52(Md61SecRwLtStLgrstInwdOtwdTrgtPosCalib_TrgtPosArray_read)
  Md62SecRwLtStLgrstUpwdDnwdTrgtPosCalib_TrgtPosArray_read/1 -> Subsystem/53(Md61SecRwLtStLgrstUpwdDnwdTrgtPosCalib_TrgtPosArray_read)
  Md62SecRwRtStBkReclnTrgtPosCalib_TrgtPosArray_read/1 -> Subsystem/54(Md61SecRwRtStBkReclnTrgtPosCalib_TrgtPosArray_read)
  Md62SecRwRtStCushFrntTrgtPosCalib_TrgtPosArray_read/1 -> Subsystem/55(Md61SecRwRtStCushFrntTrgtPosCalib_TrgtPosArray_read)
  Md62SecRwRtStLgrstInwdOtwdTrgtPosCalib_TrgtPosArray_read/1 -> Subsystem/56(Md61SecRwRtStLgrstInwdOtwdTrgtPosCalib_TrgtPosArray_read)
  Md62SecRwRtStLgrstUpwdDnwdTrgtPosCalib_TrgtPosArray_read/1 -> Subsystem/57(Md61SecRwRtStLgrstUpwdDnwdTrgtPosCalib_TrgtPosArray_read)

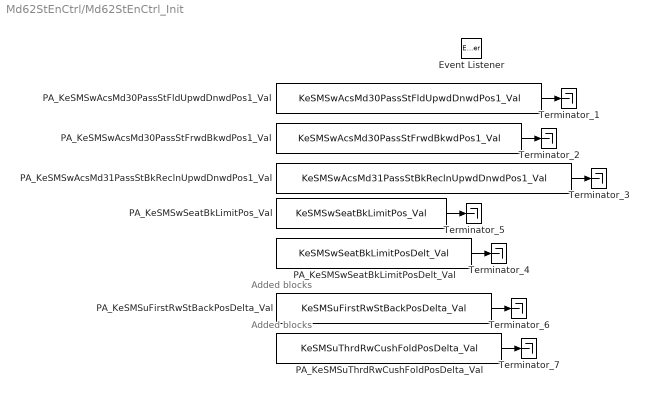
== system Md62StEnCtrl/Md62StEnCtrl_Init ==
  note: Added blocks
  note: Added blocks
  Event Listener : EventListener  EventName=reset
  PA_KeSMSuFirstRwStBackPosDelta_Val : Constant  Value=KeSMSuFirstRwStBackPosDelta_Val
  PA_KeSMSuThrdRwCushFoldPosDelta_Val : Constant  Value=KeSMSuThrdRwCushFoldPosDelta_Val
  PA_KeSMSwAcsMd30PassStFldUpwdDnwdPos1_Val : Constant  Value=KeSMSwAcsMd30PassStFldUpwdDnwdPos1_Val
  PA_KeSMSwAcsMd30PassStFrwdBkwdPos1_Val : Constant  Value=KeSMSwAcsMd30PassStFrwdBkwdPos1_Val
  PA_KeSMSwAcsMd31PassStBkReclnUpwdDnwdPos1_Val : Constant  Value=KeSMSwAcsMd31PassStBkReclnUpwdDnwdPos1_Val
  PA_KeSMSwSeatBkLimitPosDelt_Val : Constant  Value=KeSMSwSeatBkLimitPosDelt_Val
  PA_KeSMSwSeatBkLimitPos_Val : Constant  Value=KeSMSwSeatBkLimitPos_Val
  Terminator_{1..7} (7 alike) : Terminator
  wires:
  PA_KeSMSwAcsMd30PassStFldUpwdDnwdPos1_Val/1 -> Terminator_1/1
  PA_KeSMSwAcsMd30PassStFrwdBkwdPos1_Val/1 -> Terminator_2/1
  PA_KeSMSwAcsMd31PassStBkReclnUpwdDnwdPos1_Val/1 -> Terminator_3/1
  PA_KeSMSwSeatBkLimitPosDelt_Val/1 -> Terminator_4/1
  PA_KeSMSwSeatBkLimitPos_Val/1 -> Terminator_5/1
  PA_KeSMSuFirstRwStBackPosDelta_Val/1 -> Terminator_6/1
  PA_KeSMSuThrdRwCushFoldPosDelta_Val/1 -> Terminator_7/1
